simulink model "dami"  (R2020b)
settings: Solver=VariableStepAuto  StartTime=0.0  StopTime=10.0  RelTol=1e-3
settings Model: Creator=99003759  LastModifiedBy=99003759

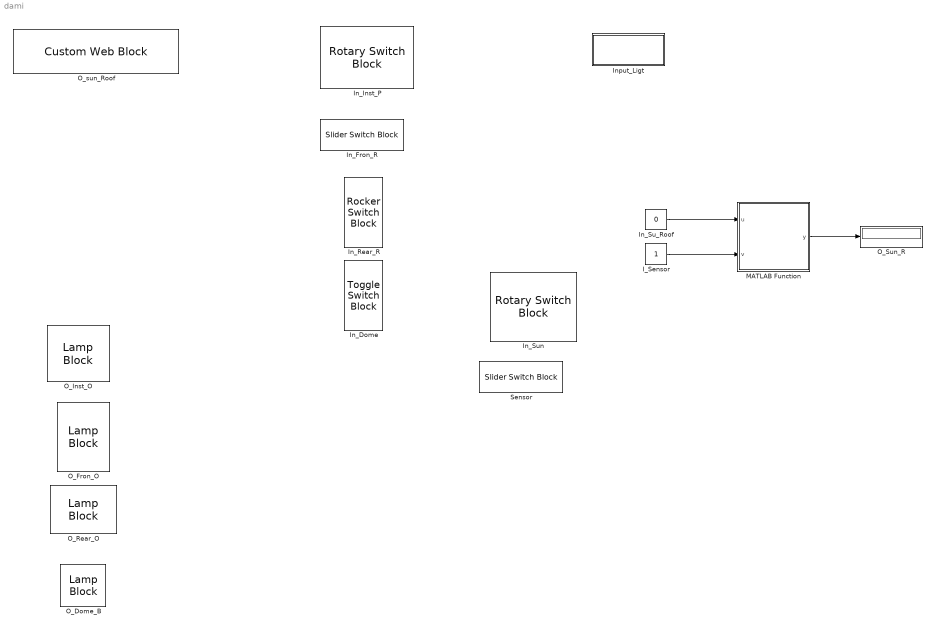
== system dami ==
  I_Sensor : Constant
  In_Dome : ToggleSwitchBlock
      settings: Values={{'Off', 'On'}, [0 1]}
  In_Fron_R : SliderSwitchBlock
      settings: Values={{'Off', 'On'}, [0 1]}
  In_Inst_P : RotarySwitchBlock
      settings: Values={{'O', 'P++,--', 'P++,--'}, [0 1 2]}
  In_Rear_R : RockerSwitchBlock
      settings: Values={{'Off', 'On'}, [0 1]}
  In_Su_Roof : Constant  Value=0
  In_Sun : RotarySwitchBlock
      settings: Values={{'No', 'P++,--', 'P++,--', 'P++,--'}, [0 1 2 3]}
  Input_Ligt : Subsystem
  MATLAB Function : MATLAB Function  TreatAsAtomicUnit=on
  O_Dome_B : LampBlock
  O_Fron_O : LampBlock
  O_Inst_O : LampBlock
  O_Rear_O : LampBlock
  O_Sun_R : Display
  O_sun_Roof : CustomWebBlock  ShowInitialText=on  Configuration="{\"components\":[{\"name\":\"LinearScaleComponent\",\"settings\":{\"bounds\":{\"max\":15,\"min\":0,\"tickInterval\":\"auto\"},\"internalTickHeightScaleFactor\":0.5,\"labelColor\":[250,245,199],\"labelFont\":{\"font\":\"Arial\",\"fontSize\":12},\"labelTransparency\":1,\"needleImage\":{\"size\":[21,75],\"src\":\"data:image\\/svg+xml;base64,PHN2ZyB4bWxucz0iaHR0cDovL3d3dy53My5vcmcvMjAwMC9zdmciIHhtbG5zOnhsaW5rPSJodHRwOi8vd3d3LnczLm9yZy8xOTk5L3hsaW5rIiB2aWV3Qm94PSIwIDAgMjEgNzUiPjxkZWZzPjxzdHlsZT4uY2xzLTF7ZmlsbDpub25lO30uY2xzLTJ7aXNvbGF0aW9uOmlzb2xhdGU7fS5jbHMtM3tjbGlwLXBhdGg6dXJsKCNjbGlwLXBhdGgpO30uY2xzLTR7b3BhY2l0eTowLjM7bWl4LWJsZW5kLW1vZGU6bXVsdGlwbHk7fS5jbHMtNXtmaWxsOiNlYjI2Mjk7fTwvc3R5bGU+PGNsaXBQYXRoIGlkPSJjbGlwLXBhdGgiIHRyYW5zZm9y ...(+1928 chars)\",\"srcOrientation\":\"horizontal\"},\"needleOffset\":[0,0.01094391244870041],\"needleSize\":{\"height\":0.7589285714285714,\"width\":0.11960078534031414},\"position\":[0.06986607142857143,0.01995798319327731,0.9641544117647058,0.8],\"scaleColors\":[{\"color\":[0,114,189],\"max\":10,\"min\":1}],\"scaleColorsSize\":0.2,\"showLabels\":1,\"showMinorTicks\":0,\"showSpanLine\":1,\"showTicks\":1,\"tickColor\":[250,245,200],\"tickTransparency\":1,\"valueBarColor\":[23,89,176],\"valueBarOffset\":0,\"valueBarSize\":0.23,\"valueBarTransparency\":1}},{\"name\":\"BackgroundImageComponent\",\"settings\":{\"image\":{\"size\":[380,101],\"src\":\"data:image\\/svg+xml;base64,PHN2ZyB4bWxucz0iaHR0cDovL3d3dy53My5vcmcvMjAwMC9zdmciIHZpZXdCb3g9IjAgMCAzODAgMTAxIj48ZGVmcz48c3R5bGU+LmNscy0xe2ZpbGw6IzAwMmI0Mjt9LmNscy0ye2ZpbGw6IzQyNzA4Mjt9LmNscy0ze2ZpbGw6IzdjYTBiMjt9PC9zdHlsZT48L2RlZnM+PHRpdGxlPmhvcml6b250YWxfZ2F1Z2VfIGJhY2tncm91bmQ8L3RpdGxlPjxnIGlkPSJMYXllcl8yIiBkYXRhLW5hbWU9IkxheWVyIDIiPjxnIGlkPSJMYXllcl8xLTIiIGRhdGEtbmFtZT0iTGF5ZXIgMSI+PHJlY3QgY2xhc3M9ImNscy0xIiB4PSIxMSIgeT0iMTEiIHdpZHRoPSIzNTgiIGhlaWdodD0iNzkiLz48cGF0aCBjbGFzcz0iY2xzLTIiIGQ9Ik04LDhWOTNIMzcyVjhaTTM2OSw5MEgxMVYxMUgzNjlaIi8+PHBhdGggY2xhc3M9ImNscy0zIiBkPSJNMCwwVjEwMUgzODBWMFpNMzcyLDkzSDhWOEgzNzJaIi8+PC9nPjwvZz48L3N2Zz4=\",\"srcOrientation\":\"horizontal\"},\"position\":[0,0,1,1],\"scaleMode\":\"0\"}},{\"name\":\"ForegroundImageComponent\",\"settings\":{\"image\":{\"size\":[0,0],\"src\":\"default\",\"srcOrientation\":[]},\"isForeground\":1,\"position\":[0,0,1,1],\"scaleMode\":\"0\"}}],\"settings\":{\"BindingType\":\"signal\",\"aspectRatio\":3.7777777777777777,\"fixedAspectRatio\":\"on\",\"orientation\":\"horizontal\"},\"type\":\"LinearGauge\"}"
  Sensor : SliderSwitchBlock
      settings: Values={{'N_Se', 'Se'}, [0 1]}
  wires:
  In_Su_Roof/1 -> MATLAB Function/1(u)
  MATLAB Function/1(y) -> O_Sun_R/1
  I_Sensor/1 -> MATLAB Function/2(v)

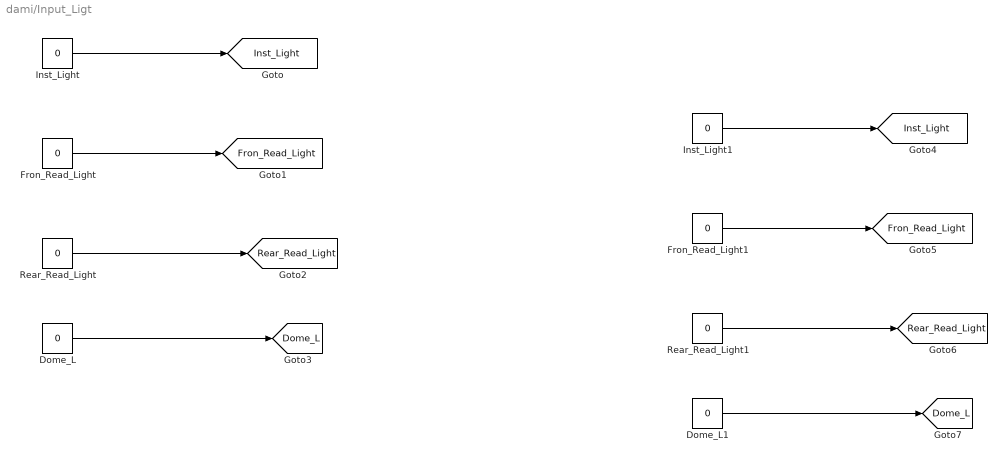
== system dami/Input_Ligt ==
  Dome_L : Constant  Value=0
  Dome_L1 : Constant  Value=0
  Fron_Read_Light : Constant  Value=0
  Fron_Read_Light1 : Constant  Value=0
  Inst_Light : Constant  Value=0
  Inst_Light1 : Constant  Value=0
  Rear_Read_Light : Constant  Value=0
  Rear_Read_Light1 : Constant  Value=0
  tag scope: Dome_L=global, Fron_Read_Light=global, Inst_Light=global, Rear_Read_Light=global
  wires:
  Inst_Light/1 -> [Inst_Light]
  Fron_Read_Light/1 -> [Fron_Read_Light]
  Rear_Read_Light/1 -> [Rear_Read_Light]
  Dome_L/1 -> [Dome_L]
  Dome_L1/1 -> [Dome_L]
  Inst_Light1/1 -> [Inst_Light]
  Fron_Read_Light1/1 -> [Fron_Read_Light]
  Rear_Read_Light1/1 -> [Rear_Read_Light]

== matlab function dami/MATLAB Function ==
  data: u input; y output; v input
function y = fcn(u,v)
if u == 1
    for i = 1:5
        y = u * i;
    end
elseif u == 2
    for i = 1:5
        y = u * i;
    end
elseif u == 3
    for i = 1:5
        y = u * i;
    end
else
    y = u;
end
if v == 1 && u ~= 0
   y = 15;
end
